simulink model "V2X_Core_SRI_coding_rate_symbol"  (R2023b)
settings: Solver=ode23tb  StartTime=0.0  StopTime=50  MaxStep=1e-2  RelTol=1e-3  AbsTol=1e-3
StopFcn:
  | run('saving.m')
values from neighbouring files (symbols this model uses):
  b = 1.6    [a2024_v2x_matlab_6veh.m]
  m = 2000    [a2024_v2x_matlab_6veh.m]
  mEgo = 1500    [a2024_v2x_matlab_6veh.m]
  Mode = 1    [a2024_v2x_matlab_6veh.m]    (also in v2x_matlab.m; v2x_matlabV2.m; v2x_matlab_6veh.m; v2x_matlab_R.m)
  RefSpeed = 90/3.6    (= 25)    [v2x_matlabV2.m]    (also in v2x_matlab_R.m)
  RelDistThreshold = 300    [v2x_matlabV2.m]    (also in v2x_matlab_R.m)
  s = RandStream("dsfmt19937","Seed",15)    [v2x_matlab.m]
  sampleTime = 0.1    [a2024_v2x_matlab_6veh.m]    (also in v2x_matlab.m; v2x_matlabV2.m; v2x_matlab_6veh.m; v2x_matlab_R.m)
  waypoints = [egoWP(:,2) egoWP(:,1), zeroforwp]    [a2024_v2x_matlab_6veh.m]    (also in misc.m = data.data.ActorSpecifications(1,1).Waypoints(:,[1,2]); v2x_matlab.m = data.data.ActorSpecifications(1,1).Waypoints(:,[1,2]); v2x_matlabV2.m = [5 -1.6 0; v2x_matlab_R.m = [5 -1.6 0)
  ZeroActors = struct(     'ActorID',0,     'Position', [1000 1000 1000],      'Velocity', [0 0 0],      'Roll', 0,      'Pitch', 0,      'Yaw', 0,      'AngularVelocity', [0 0 0])    [v2x_matlabV2.m]    (also in v2x_matlab_R.m)
undefined symbols (not defined in the file or in its folder): Battery, Brakes, Control, DiscIntNeverNeededParam, doppler, Drivetrain, ElectricMotor, Env, FB_flag, Init, SNR_value_list, Vehicle, Wheels
libraries: simulink x45, commofdm x29, commdigbbndam3 x15, commchan3 x14, simulink_extras x13, commcnvcod2 x12, commdigbbndpm3 x11, commblkintrlv2 x10, dspmathops x6, sharedtransform x6, autolibutils x6, autolibsharedcoupling x4
(part 7 of 8)

== matlab function V2X_Core_SRI_coding_rate_symbol/Subsystem2/MATLAB Function1 ==
  data: busActors3Test1 input; Actor output int16 size=15; VehicleID input; VehicleData output Bus: Actors; EgoData input Bus: Actors; counter output
  events: trigger input RISING_EDGE_EVENT
function [Actor, VehicleData, counter]  = convBus2IntVector(busActors3Test1, VehicleID, EgoData)

% Data extracted from actorss bus

%ActorId = BusActors1Actors.Actors(ActorID).ActorID(1:1);
numActors = busActors3Test1.NumActors;
%time = busActors3Test1.Time;
time = busActors3Test1.Time;

ActorID = VehicleID;

posX = busActors3Test1.Actors(ActorID).Position(1:1);
posY = busActors3Test1.Actors(ActorID).Position(2:2);
posZ = busActors3Test1.Actors(ActorID).Position(3:3);
vPos = [posX posY posZ];

vX = busActors3Test1.Actors(ActorID).Velocity(1:1);
vY = busActors3Test1.Actors(ActorID).Velocity(2:2);
vZ = busActors3Test1.Actors(ActorID).Velocity(3:3);

roll = busActors3Test1.Actors(ActorID).Roll(1:1);
pitch = busActors3Test1.Actors(ActorID).Pitch(1:1);
yaw = busActors3Test1.Actors(ActorID).Yaw(1:1);


angularVelocityX = busActors3Test1.Actors(ActorID).AngularVelocity(1:1);
angularVelocityY = busActors3Test1.Actors(ActorID).AngularVelocity(2:2);
angularVelocityZ = busActors3Test1.Actors(ActorID).AngularVelocity(3:3);

VehicleData = busActors3Test1.Actors(ActorID);


%% Converting the data

ActorID = int16(ActorID);

posMultip = 10;
posX = int16(round(posMultip*posX));
posY = int16(round(posMultip*posY));
posZ = int16(round(posMultip*posZ));

velMultip = 50;
vX = int16(round(velMultip * vX));
vY = int16(round(velMultip * vY));
vZ = int16(round(velMultip * vZ));

rpyMultip = 50;
roll = int16(round(rpyMultip * roll));
pitch = int16(round(rpyMultip * pitch));
yaw = int16(round(rpyMultip * yaw));

angvelMultip = 50;
angularVelocityX = int16(round(angvelMultip * angularVelocityX));
angularVelocityY = int16(round(angvelMultip * angularVelocityY));
angularVelocityZ = int16(round(angvelMultip * angularVelocityZ));


% Output vector
%zerosVector = zeros(9,1);

intVector = [numActors; time; ActorID; posX; posY; posZ; vX; vY; vZ; roll; pitch; yaw; angularVelocityX; angularVelocityY; angularVelocityZ];



%% Pathloss (freespace)

EgoPos = EgoData.Position;
dist = norm(vPos - EgoPos);

fc = 5.9*10^9;  % Carrier frequency
lambda = physconst('LightSpeed')/fc;

PL = fspl(dist, lambda);

Pt_dBm = 33;    % [dBm] Transmission power; maximum permissible transmit power level
sigma = rand(1) + 3.2;  % [3.7 +- 0.5] Variance of the shadowing effect in the wireless communication channel
                        % shadowing follows a log-normal random distribution
X = randn(1);       % random variable following a normal distribution with mean 0 and standard deviation 1
SH = sigma * X;

Pr = Pt_dBm - PL - SH;

P_SEN = -40;

ZeroActors = int16(zeros(15,1));

persistent prev_value;
if isempty(prev_value)
    prev_value = ZeroActors; % Initialize to a default value
end

if Pr > P_SEN
    Actor = intVector;
    prev_value = intVector;
else
    Actor = prev_value;
end


%% Packet counter
counter = 0;

if (Pr > P_SEN)
    counter = counter + 1;
end


end

== matlab function V2X_Core_SRI_coding_rate_symbol/VehicleDynamic/MATLAB Function1 ==
  data: RefSpeed input; RefSpeedMax output size=1; v_HV input; v_RV input; pdr input; lat input; sri_target input; sri_val output; RelDist input; Headway output
function [RefSpeedMax, sri_val, Headway] = calculate_SRI_max_speed(RefSpeed, v_HV, v_RV, pdr, lat, sri_target, RelDist)

    %V_HV_UPPER_LIMIT = 1.0
    %V_HV_LOWER_LIMIT = 0.0
    % SRI_TARGET = 0.1;
    DEFAULT_HV_SPEED = 190 / 3.6; % in m/s
    DEFAULT_RV_SPEED =  190 / 3.6; % in m/s


    pdr_normalized = pdr / 100;
    lat_normalized = lat / 1000;
    v_HV_normalized = v_HV / DEFAULT_HV_SPEED;
    v_RV_normalized = v_RV / DEFAULT_RV_SPEED;
    
    if abs(v_HV) < 0.001
        Speed_reciproc = 0;
    else
        Speed_reciproc = 1/v_HV;
    end

    Headway = RelDist*Speed_reciproc;
    if Headway > 50
        Headway = 50;
    end



    if v_RV-1 > v_HV || pdr < 0.1
        RefSpeedMax = RefSpeed;
        sri_val = -1;
    else
        sri_val = SRI_value(v_HV_normalized,v_RV_normalized, pdr_normalized, lat_normalized);
        if sri_val <= sri_target
            RefSpeedMax = RefSpeed;
        else
            lb0 = 0.0;
            ub0 = v_HV_normalized;
            x0 = 1.0;
            %value_bounds = Bounds([V_HV_LOWER_LIMIT],[v_HV_normalized])
            opts = optimoptions('fmincon','Algorithm','sqp');
            sri_err_fun = @(v_HV_norm) abs(SRI_value(v_HV_norm, v_RV_normalized, pdr_normalized, lat_normalized) - sri_target); 
            v_HV_max_normalized = fmincon(sri_err_fun, x0,[], [],[],[], lb0, ub0, [], opts);
            %res = minimize(fun=SRI_target_function, x0=[1.0], bounds=value_bounds, args=(v_RV_normalized, pdr_normalized, lat_normalized, sri_target))
            %v_HV_max_normalized = res.x[0];
            if Headway < 1.3
                RefSpeedMax = v_RV;
            else
                RefSpeedMax = v_HV_max_normalized*DEFAULT_HV_SPEED; % in m/s
            end
        end
    end

end
function sri_value = SRI_value(v_HV_norm, v_RV_norm, pdr_norm, lat_norm)

    OLSparams = [0.1283, -0.0089, -0.2621, -0.0181, 0.6640, -0.0156, -0.2030, -1.1130, 0.3615, 0.1294, 0.5597, 0.1044, 0.0613, -0.5524, 0.0934];
    sri_value =   OLSparams(1) ...
                + OLSparams(2)  * v_HV_norm ...
                + OLSparams(3)  * v_RV_norm ...
                + OLSparams(4)  * pdr_norm ...
                + OLSparams(5)  * v_HV_norm^2 ...
                + OLSparams(6)  * v_RV_norm^2 ...
                + OLSparams(7)  * v_RV_norm * pdr_norm ...
                + OLSparams(8)  * pdr_norm * (v_HV_norm^2) ...
                + OLSparams(9)  * pdr_norm * (v_RV_norm^2) ...
                + OLSparams(10) * lat_norm * (v_HV_norm^2) ...
                + OLSparams(11) * (v_HV_norm^2) * (pdr_norm^2) ...
                + OLSparams(12) * v_HV_norm * v_RV_norm * lat_norm ...
                + OLSparams(13) * v_RV_norm * pdr_norm * lat_norm ...
                + OLSparams(14) * v_RV_norm * lat_norm * (v_HV_norm^2)...
                + OLSparams(15) * lat_norm * (v_HV_norm^2) * (v_RV_norm^2);
end


% % 
% % v_HV_0 = 0.0;
% % SRI_target = 0.5;
% % v_RV = v_RV_original / (50.0/3.6);
% % 
% % OLSparams = [0.1283, -0.0089, -0.2621, -0.0181, 0.6640, -0.0156, -0.2030, -1.1130, 0.3615, 0.1294, 0.5597, 0.1044, 0.0613, -0.5524, 0.0934];
% % 
% % 
% % SRI = @(v_HV) abs(OLSparams(1) ...
% %                 + OLSparams(2) * PDR ...
% %                 + OLSparams(3) * LAT ...
% %                 + OLSparams(4) * v_HV ...
% %                 + OLSparams(5) * v_HV^2 ...
% %                 + OLSparams(6) * PDR * v_HV ...
% %                 + OLSparams(7) * PDR * v_RV ...
% %                 + OLSparams(8) * v_HV * v_RV^2 ...
% %                 + OLSparams(9) * v_RV * v_HV^2 ...
% %                 + OLSparams(10) * PDR * v_RV * v_HV^2 ...
% %                 + OLSparams(11) * PDR^2 * v_HV * v_RV^2 ...
% %                 + OLSparams(12) * PDR^2 * v_HV^2 * v_RV ...
% %                 + OLSparams(13) * PDR^2 * v_HV^2*v_RV^2 ...
% %                 - SRI_target);
% %  v_HV = fminsearch(SRI, v_HV_0) * 130.0/3.6;
% % end

== matlab function V2X_Core_SRI_coding_rate_symbol/DSRC/Subsystem3/3//4 64 QAM/MATLAB Function3 ==
  settings: updateMethod=DISCRETE
  data: input input; output output
function output = removeZeros(input)

output = input(1:40,:,:);

end

== matlab function V2X_Core_SRI_coding_rate_symbol/DSRC/Subsystem4/MATLAB Function1 ==
  settings: sampleTime=inherited
  data: busActors3Test1 input; Actor output int16 size=15; VehicleID input; VehicleData output Bus: Actors; EgoData input Bus: Actors; counter_out output; SNR output; Pr output
  events: trigger input RISING_EDGE_EVENT
function [Actor, VehicleData, counter_out, SNR, Pr]  = convBus2IntVector(busActors3Test1, VehicleID, EgoData)

% Data extracted from actorss bus

%ActorId = BusActors1Actors.Actors(ActorID).ActorID(1:1);
numActors = busActors3Test1.NumActors;
%time = busActors3Test1.Time;
time = busActors3Test1.Time;

ActorID = VehicleID;

posX = busActors3Test1.Actors(ActorID).Position(1:1);
posY = busActors3Test1.Actors(ActorID).Position(2:2);
posZ = busActors3Test1.Actors(ActorID).Position(3:3);
vPos = [posX posY posZ];

vX = busActors3Test1.Actors(ActorID).Velocity(1:1);
vY = busActors3Test1.Actors(ActorID).Velocity(2:2);
vZ = busActors3Test1.Actors(ActorID).Velocity(3:3);

roll = busActors3Test1.Actors(ActorID).Roll(1:1);
pitch = busActors3Test1.Actors(ActorID).Pitch(1:1);
yaw = busActors3Test1.Actors(ActorID).Yaw(1:1);


angularVelocityX = busActors3Test1.Actors(ActorID).AngularVelocity(1:1);
angularVelocityY = busActors3Test1.Actors(ActorID).AngularVelocity(2:2);
angularVelocityZ = busActors3Test1.Actors(ActorID).AngularVelocity(3:3);

VehicleData = busActors3Test1.Actors(VehicleID);


%% Converting the data

ActorID = int16(ActorID);

posMultip = 10;
posX = int16(round(posMultip*posX));
posY = int16(round(posMultip*posY));
posZ = int16(round(posMultip*posZ));

velMultip = 50;
vX = int16(round(velMultip * vX));
vY = int16(round(velMultip * vY));
vZ = int16(round(velMultip * vZ));

rpyMultip = 50;
roll = int16(round(rpyMultip * roll));
pitch = int16(round(rpyMultip * pitch));
yaw = int16(round(rpyMultip * yaw));

angvelMultip = 50;
angularVelocityX = int16(round(angvelMultip * angularVelocityX));
angularVelocityY = int16(round(angvelMultip * angularVelocityY));
angularVelocityZ = int16(round(angvelMultip * angularVelocityZ));


% Output vector
%zerosVector = zeros(9,1);

intVector = [numActors; time; ActorID; posX; posY; posZ; vX; vY; vZ; roll; pitch; yaw; angularVelocityX; angularVelocityY; angularVelocityZ];


%% Pathloss (freespace)

EgoPos = EgoData.Position;
dist = norm(vPos - EgoPos);

fc = 5.9e9;  % Carrier frequency
lambda = (physconst('LightSpeed'))/fc;

PL = fspl(dist, lambda);

Pt_dBm = 33;    % [dBm] Transmission power; maximum permissible transmit power level
Pt_dbW = Pt_dBm - 30;
sigma = rand(1) + 3.2;  % [3.7 +- 0.5] Variance of the shadowing effect in the wireless communication channel
                        % shadowing follows a log-normal random distribution
X = 2*rand(1)-1;      % random variable following a normal distribution with mean 0 and standard deviation 1
SH = sigma * X;

% h_T = 1;
% h_R = 1;
% dF =  (4*h_T*h_R)/lambda
% lambda1 = 1.61; % Pathloss exponent LOS
% lambda2 = 1.85; % Pathloss exponent NLOS

Pr = Pt_dBm - PL - SH; 

% l1 = 10*lambda1*log(dF)
% l2 = 10*lambda2*log(dist/dF)
% Pr = Prt - l1 - l2 + SH;

P_SEN = -60;

%ZeroActors = int16(zeros(15,1));
% 
% counter = 0;
% storedPacket = int16(nan(15,1));
% 
% if Pr > P_SEN
%     Actor = intVector;
%     storedPacket = intVector;
%     counter = 0;
% elseif counter < 10
%     Actor = storedPacket;
%     counter = counter + 1;
% end


%disp(storedPacket)


% persistent prev_value;
% if isempty(prev_value)
%     prev_value = int16(nan(15,1)); % Initialize to a default value
% end
% 
% if Pr > P_SEN
%     Actor = intVector;
%     prev_value = intVector;
%     counter = 0;
% elseif counter < 1
%     Actor = prev_value;
%     counter = counter + 1;
% end

Actor = intVector;
%% SNR
bandwidth = 10e6;
F = 6; % [dB] Noise figure
k = physconst('Boltzmann'); % Boltzmann állandó
T = 300; % [K] Abszolút hőmérséklet

N0 = bandwidth *k*T;
N0dbm = 10 * log10(1000*N0);
N0dbW = N0dbm - 30; 
%N0 = -99;
SNR = Pr - N0dbm;
%signalpower = Pr;s


%% Packet counter
persistent counter
if isempty(counter)
    counter = 0;
end

if (Pr > P_SEN)
    counter = counter + 1;
end

counter_out = counter;
end

== matlab function V2X_Core_SRI_coding_rate_symbol/DSRC/Subsystem4/MATLAB Function2 ==
  settings: updateMethod=DISCRETE  sampleTime=sampleTime
  data: modulated input; signal output; SNR input
function signal = PRO_error(modulated, SNR)

signal = awgn(modulated,SNR);

== matlab function V2X_Core_SRI_coding_rate_symbol/Channel/MATLAB Function1 ==
  data: Actors output Bus: Actors; ActorsIn input; Positions output; Distances output; Ego input
function [Actors, Positions, Distances] = SelectActor(ActorsIn, Ego)

EgoActor = Ego;
Actors = ActorsIn.Actors;


% Separating
Lead = ActorsIn.Actors(1);
Interfering = ActorsIn.Actors(3);
Threshold = ActorsIn.Actors(2);

% Distances
EgoPos = Ego.Position';
LeadPos = Lead.Position';
InterferingPos = Interfering.Position';
ThresholdPos = Threshold.Position';

Positions = [EgoPos LeadPos InterferingPos ThresholdPos];

%EgoDists
EgoDist = [norm(EgoPos-EgoPos);
            norm(EgoPos-LeadPos);
            norm(EgoPos-InterferingPos);
            norm(EgoPos-ThresholdPos)];

%LeadDists
LeadDist = [norm(LeadPos-EgoPos);
            norm(LeadPos-LeadPos);
            norm(LeadPos-InterferingPos);
            norm(LeadPos-ThresholdPos)];

%InterferringDists
InterferringDist = [norm(InterferingPos-EgoPos);
                    norm(InterferingPos-LeadPos);
                    norm(InterferingPos-InterferingPos);
                    norm(InterferingPos-ThresholdPos)];

% ThresholdDists
ThresholdDist = [norm(ThresholdPos-EgoPos);
                norm(ThresholdPos-LeadPos);
                norm(ThresholdPos-InterferingPos);
                norm(ThresholdPos-ThresholdPos)];


Distances = [EgoDist, LeadDist, InterferringDist, ThresholdDist] ;

end

== matlab function V2X_Core_SRI_coding_rate_symbol/DSRC/Subsystem5/MATLAB Function1 ==
  settings: sampleTime=inherited
  data: busActors3Test1 input; Actor output int16 size=15; VehicleID input; VehicleData output Bus: Actors; EgoData input Bus: Actors; counter_out output; SNR output; Pr output
  events: trigger input RISING_EDGE_EVENT
function [Actor, VehicleData, counter_out, SNR, Pr]  = convBus2IntVector(busActors3Test1, VehicleID, EgoData)

% Data extracted from actorss bus

%ActorId = BusActors1Actors.Actors(ActorID).ActorID(1:1);
numActors = busActors3Test1.NumActors;
%time = busActors3Test1.Time;
time = busActors3Test1.Time;

ActorID = VehicleID;

posX = busActors3Test1.Actors(ActorID).Position(1:1);
posY = busActors3Test1.Actors(ActorID).Position(2:2);
posZ = busActors3Test1.Actors(ActorID).Position(3:3);
vPos = [posX posY posZ];

vX = busActors3Test1.Actors(ActorID).Velocity(1:1);
vY = busActors3Test1.Actors(ActorID).Velocity(2:2);
vZ = busActors3Test1.Actors(ActorID).Velocity(3:3);

roll = busActors3Test1.Actors(ActorID).Roll(1:1);
pitch = busActors3Test1.Actors(ActorID).Pitch(1:1);
yaw = busActors3Test1.Actors(ActorID).Yaw(1:1);


angularVelocityX = busActors3Test1.Actors(ActorID).AngularVelocity(1:1);
angularVelocityY = busActors3Test1.Actors(ActorID).AngularVelocity(2:2);
angularVelocityZ = busActors3Test1.Actors(ActorID).AngularVelocity(3:3);

VehicleData = busActors3Test1.Actors(VehicleID);


%% Converting the data

ActorID = int16(ActorID);

posMultip = 10;
posX = int16(round(posMultip*posX));
posY = int16(round(posMultip*posY));
posZ = int16(round(posMultip*posZ));

velMultip = 50;
vX = int16(round(velMultip * vX));
vY = int16(round(velMultip * vY));
vZ = int16(round(velMultip * vZ));

rpyMultip = 50;
roll = int16(round(rpyMultip * roll));
pitch = int16(round(rpyMultip * pitch));
yaw = int16(round(rpyMultip * yaw));

angvelMultip = 50;
angularVelocityX = int16(round(angvelMultip * angularVelocityX));
angularVelocityY = int16(round(angvelMultip * angularVelocityY));
angularVelocityZ = int16(round(angvelMultip * angularVelocityZ));


% Output vector
%zerosVector = zeros(9,1);

intVector = [numActors; time; ActorID; posX; posY; posZ; vX; vY; vZ; roll; pitch; yaw; angularVelocityX; angularVelocityY; angularVelocityZ];


%% Pathloss (freespace)

EgoPos = EgoData.Position;
dist = norm(vPos - EgoPos);

fc = 5.9e9;  % Carrier frequency
lambda = (physconst('LightSpeed'))/fc;

PL = fspl(dist, lambda);

Pt_dBm = 33;    % [dBm] Transmission power; maximum permissible transmit power level
Pt_dbW = Pt_dBm - 30;
sigma = rand(1) + 3.2;  % [3.7 +- 0.5] Variance of the shadowing effect in the wireless communication channel
                        % shadowing follows a log-normal random distribution
X = 2*rand(1)-1;      % random variable following a normal distribution with mean 0 and standard deviation 1
SH = sigma * X;

% h_T = 1;
% h_R = 1;
% dF =  (4*h_T*h_R)/lambda
% lambda1 = 1.61; % Pathloss exponent LOS
% lambda2 = 1.85; % Pathloss exponent NLOS

Pr = Pt_dBm - PL - SH; 

% l1 = 10*lambda1*log(dF)
% l2 = 10*lambda2*log(dist/dF)
% Pr = Prt - l1 - l2 + SH;

P_SEN = -60;

%ZeroActors = int16(zeros(15,1));
% 
% counter = 0;
% storedPacket = int16(nan(15,1));
% 
% if Pr > P_SEN
%     Actor = intVector;
%     storedPacket = intVector;
%     counter = 0;
% elseif counter < 10
%     Actor = storedPacket;
%     counter = counter + 1;
% end


%disp(storedPacket)


% persistent prev_value;
% if isempty(prev_value)
%     prev_value = int16(nan(15,1)); % Initialize to a default value
% end
% 
% if Pr > P_SEN
%     Actor = intVector;
%     prev_value = intVector;
%     counter = 0;
% elseif counter < 1
%     Actor = prev_value;
%     counter = counter + 1;
% end

Actor = intVector;
%% SNR
bandwidth = 10e6;
F = 6; % [dB] Noise figure
k = physconst('Boltzmann'); % Boltzmann állandó
T = 300; % [K] Abszolút hőmérséklet

N0 = bandwidth *k*T;
N0dbm = 10 * log10(1000*N0);
N0dbW = N0dbm - 30; 
%N0 = -99;
SNR = Pr - N0dbm;
%signalpower = Pr;s


%% Packet counter
persistent counter
if isempty(counter)
    counter = 0;
end

if (Pr > P_SEN)
    counter = counter + 1;
end

counter_out = counter;
end

== matlab function V2X_Core_SRI_coding_rate_symbol/DSRC/Subsystem5/MATLAB Function2 ==
  settings: updateMethod=DISCRETE  sampleTime=sampleTime
  data: modulated input; signal output; SNR input
function signal = PRO_error(modulated, SNR)

signal = awgn(modulated,SNR);

== matlab function V2X_Core_SRI_coding_rate_symbol/Channel/MATLAB Function9 ==
  data: Ego input; Actors input Bus: Actors; LeadActor output Bus: Actors size=1; InterferingActor output Bus: Actors size=1; ThresholdActor output Bus: Actors size=1; PSR output; Positions input; ZeroActors input
function [LeadActor,InterferingActor,ThresholdActor,PSR] = SEN_PSR(Ego, Actors, Positions, ZeroActors)
coder.extrinsic('Simulink.Bus')

%% Extract data
Lead = Actors(1);
Interfering = Actors(2);
Threshold = Actors(3);

EgoPos = Positions(:,1);
LeadPos = Positions(:,2);
InterferingPos = Positions(:,3);
ThresholdPos = Positions(:,4);

%% Calculating distances
de_lead = norm(LeadPos - EgoPos);                % Ego-Lead Distance
de_interfering = norm(InterferingPos - EgoPos);  % Ego-Interferring Distance
de_threshold = norm(ThresholdPos  - EgoPos);     % Ego-Threshold distance

dl_interfering = norm(InterferingPos - LeadPos);
dl_threshold = norm(ThresholdPos - LeadPos);

di_threshold = norm(ThresholdPos - InterferingPos);

%% Pathloss (freespace)
fc = 5.9*10^9;  % Carrier frequency
lambda = physconst('LightSpeed')/fc;

PL_EL = fspl(de_lead, lambda);
PL_EI = fspl(de_interfering, lambda);
PL_ET = fspl(de_threshold, lambda);

PL_LI = fspl(dl_interfering, lambda);
PL_LT = fspl(dl_threshold, lambda);

PL_IT = fspl(di_threshold, lambda);


% Transmission Power (Pt)
Pt_dBm = 33;    % [dBm] Transmission power; maximum permissible transmit power level
%Pt_dBw = Pt_dBm - 30; % [dBw]
%Pt_watts = (10 .^ (dBm / 10))/1000;  % Transmission power in W

sigma = rand(1) + 3.2;  % [3.7 +- 0.5] Variance of the shadowing effect in the wireless communication channel
                        % shadowing follows a log-normal random distribution
X = randn(1);       % random variable following a normal distribution with mean 0 and standard deviation 1
SH = sigma * X;
Pr_EL = Pt_dBm - PL_EL - SH; 
Pr_EI = Pt_dBm - PL_EI - SH;
Pr_ET = Pt_dBm - PL_ET - SH;

Pr_LI = Pt_dBm - PL_LI  - SH;
Pr_LT = Pt_dBm - PL_LT  - SH;

Pr_IT = Pt_dBm - PL_IT  - SH;


P_SEN = -60;  % [dBm] Sensing threshold
% P_SEN_dBW = P_SEN + 30;

% Lead
persistent prev_value_lead;
if isempty(prev_value_lead)
    prev_value_lead = ZeroActors; % Initialize to a default value
end

if Pr_EL > P_SEN
    LeadActor = Lead;
    prev_value_lead = Lead;
else
    LeadActor = prev_value_lead;
end

% Interfering
%InterferingActorOut = struct;

persistent prev_value_int;
if isempty(prev_value_int)
    prev_value_int = ZeroActors; % Initialize to a default value
end

if Pr_EI > P_SEN
    InterferingActor = Interfering;
    prev_value_int = Interfering;
else
    InterferingActor = prev_value_int;
end

% Threshold
persistent prev_value_thr;


if isempty(prev_value_thr)
    prev_value_thr = ZeroActors; % Initialize to a default value
end

if Pr_ET > P_SEN
    ThresholdActor = Threshold;
    prev_value_thr = Threshold;
else
    ThresholdActor = prev_value_thr;
end


%% PSR 
sigmasqrt2 = sigma * sqrt(2);

% Ego - Lead
deltaPtSEN_EL = Pt_dBm - PL_EL - P_SEN;
delta_SEN_EL = 0.5*(1-erf(deltaPtSEN_EL/sigmasqrt2));
PSR_EL = 1-delta_SEN_EL;

% Ego - Interfering
deltaPtSEN_EI = Pt_dBm - PL_EI - P_SEN;
delta_SEN_EI = 0.5*(1-erf(deltaPtSEN_EI/sigmasqrt2));
PSR_EI = 1-delta_SEN_EI;

% Ego - Threshold
deltaPtSEN_ET = Pt_dBm - PL_ET - P_SEN;
delta_SEN_ET = 0.5*(1-erf(deltaPtSEN_ET/sigmasqrt2));
PSR_ET = 1-delta_SEN_ET;

% Lead - Interfering
deltaPtSEN_LI = Pt_dBm - PL_LI - P_SEN;
delta_SEN_LI = 0.5*(1-erf(deltaPtSEN_LI/sigmasqrt2));
PSR_LI = 1-delta_SEN_LI;

% Lead - Threshold
deltaPtSEN_LT = Pt_dBm - PL_LT - P_SEN;
delta_SEN_LT = 0.5*(1-erf(deltaPtSEN_LT/sigmasqrt2));
PSR_LT = 1-delta_SEN_LT;

% Interfering - Threshold;
deltaPtSEN_IT = Pt_dBm - PL_IT - P_SEN;
delta_SEN_IT = 0.5*(1-erf(deltaPtSEN_IT/sigmasqrt2));
PSR_IT = 1-delta_SEN_IT;


PSR = [PSR_EL PSR_EI PSR_ET PSR_LI PSR_LT PSR_IT];

end

== matlab function V2X_Core_SRI_coding_rate_symbol/Channel/MATLAB Function4 ==
  data: PSR input; CBR output
function CBR = CBR(PSR)

lambda = (1/0.01)*3;            % Packets/second
T = 0.008;                      % Packet duration


beta = 4*4.7/400;   % Traffic density (vehicle/meter)

load_ir = lambda * T * PSR;

% CBR upper bound:
CBR_u = beta * sum(load_ir);    % distance between vehicle vi and the ego vehicle
                                % upper bound, because it does not take into account packet collisions
p1 = -0.2481;
p2 = 0.913;
p3 = 0.003844;

CBR = p1*CBR_u^2 + p2*CBR_u + p3

end

== matlab function V2X_Core_SRI_coding_rate_symbol/Ego trajectory ==
  settings: updateMethod=DISCRETE  sampleTime=sampleTime
  data: EgoFdbX input; EgoFdbY input; LongRef output; LatRef output; YawRef output; waypoints input
function [LongRef, LatRef, YawRef] = generateTrajectory(EgoFdbX, EgoFdbY, waypoints)

LongFdb = EgoFdbX;
LatFdb = EgoFdbY;
EgoFdb= [LongFdb, LatFdb]; % Ego feedback positions norm

% waypoints = [-104.6000, 6.6000, deg2rad(2.9993);
%             54.7000, -14.8000, deg2rad(-29.0375);
%             91.4000, -42.6000, deg2rad(-44.2776);
%             163.6000, -148.6000, deg2rad(-61.4646)];





count = 1;

min_distance = inf;

for i = 1:size(waypoints, 1)
    RefPose = waypoints(i,1:2);
    distance = norm(RefPose - EgoFdb);

    if abs(distance) < min_distance
        min_distance = abs(distance);
        count = i;
    end
end


if count > size(waypoints, 1)
    count = size(waypoints, 1);  % Ensure count doesn't exceed the number of rows in waypoints
end


LongRef = waypoints(count,1);
LatRef = waypoints(count,2);
YawRef = waypoints(count,3);
Output = [LongRef, LatRef, YawRef];
end


% while count <= size(waypoints, 1)
%     RefPosenorm = norm(waypoints(count,1:2));
%     if EgoFdbnorm < RefPosenorm
%         break;
%     else
%         count = count + 1;
%     end
% end
% 
% if count > size(waypoints, 1)
%     count = size(waypoints, 1);  
% end
% 
% RefPose = waypoints(count,:);
% end

% if 0 <= timevector < 1
%     RefPose = waypoints(1,:);
% elseif 1 <= timevector < 2
%     RefPose = waypoints(2,:);
% elseif 2 <= timevector < 3
%     RefPose = waypoints(3,:);
% elseif 3 <= timevector < 4
%     RefPose = waypoints(4,:);
% elseif 4 <= timevector < 5
%     RefPose = waypoints(5,:);
% elseif 5 <= timevector < 6
%     RefPose = waypoints(6,:);
% elseif 6 <= timevector < 7
%     RefPose = waypoints(7,:);
% elseif 7 <= timevector < 8
%     RefPose = waypoints(8,:);
% elseif 8 <= timevector < 9
%     RefPose = waypoints(9,:);
% elseif 9 <= timevector < 10
%     RefPose = waypoints(10,:);
% elseif 10 <= timevector < 11
%     RefPose = waypoints(11,:);
% end
% 
% end

== stateflow chart V2X_Core_SRI_coding_rate_symbol/VehicleDynamic/FiveSteteABS-TCS/ABSCtrlForEach/For Each Subsystem/ABSForEachWheel ==
  state ABSOff
    entry:
    PbOutput = Pref;
    Flag = 0;
    during:
    PbOutput = Pref;
  state Normal
    entry:
    PbOutput = Pref;
    Flag = 0;
    during:
    PbOutput = Pref;
  state ABSOn
    state Phase1
      entry:
      PbOutput = v1;
      Flag = 1;
    state Phase5
      entry:
      PbOutput = v5;
      Flag = 5;
    state Phase2
      entry:
      PbOutput = 0;
      Flag = 2;
    state Phase4
      entry:
      PbOutput = 0;
      Flag = 4;
    state Phase3
      entry:
      PbOutput = v4;
      Flag = 3;
    (default) -> Phase1
    Phase5 -> Phase1 : [e2 < a2]
    Phase1 -> Phase2 : [e2 >= b]
    Phase4 -> Phase5 : [e2 <= a1]
    Phase2 -> Phase3 : [e2 >= A]
    Phase3 -> Phase4 : [e2 < A]
  (default) -> ABSOff
  ABSOn -> ABSOff : [abs(VehSpd) < 0.1 || Pref <= 0]
  Normal -> ABSOff [order 2] : [Pref <= 0]
  ABSOff -> Normal : [Pref > 0 && e2 < a2]
  Normal -> ABSOn [order 1] : [e1 < 0]
  data: e1 input; e2 input; PbOutput output; Flag output; b parameter; v1 parameter; v4 parameter; v5 parameter; A parameter; a2 parameter; a1 parameter; Pref input; VehSpd input

== stateflow chart V2X_Core_SRI_coding_rate_symbol/VehicleDynamic/FiveSteteABS-TCS/TCSCtrlForEach/For Each Subsystem/ABSForEachWheel ==
  state TCSOff
    entry:
    PbOutput = 0;
    Flag = 0;
    during:
    PbOutput = 0;
  state Normal
    entry:
    PbOutput = 0;
    Flag = 0;
    during:
    PbOutput = 0;
  state TCSOn
    state Phase1
      entry:
      PbOutput = v1;
      Flag = 1;
    state Phase5
      entry:
      PbOutput = v5;
      Flag = 5;
    state Phase2
      entry:
      PbOutput = 0;
      Flag = 2;
    state Phase4
      entry:
      PbOutput = 0;
      Flag = 4;
    state Phase3
      entry:
      PbOutput = v4;
      Flag = 3;
    (default) -> Phase1
    Phase5 -> Phase1 : [e2 > a2]
    Phase1 -> Phase2 : [e2 <= b]
    Phase4 -> Phase5 : [e2 >= a1]
    Phase2 -> Phase3 : [e2 <= A]
    Phase3 -> Phase4 : [e2 > A]
  (default) -> TCSOff
  TCSOn -> TCSOff : [Pb <= 0 || AccelFdbk <= 0.2|| e1<0.1]
  Normal -> TCSOff [order 2] : [AccelFdbk <= 0]
  TCSOff -> Normal : [AccelFdbk > 0 && e2 > a2 && Enb > 0.3]
  Normal -> TCSOn [order 1] : [e1 > 0]
  data: e1 input; e2 input; PbOutput output; Flag output; b parameter; v1 parameter; v4 parameter; v5 parameter; A parameter; a2 parameter; a1 parameter; AccelFdbk input; Enb input; Pb input

== matlab function V2X_Core_SRI_coding_rate_symbol/MATLAB Function6 ==
  settings: updateMethod=DISCRETE  sampleTime=sampleTime
  data: xdotin input; y output
function y = initialVelocity(xdotin)

if isempty(xdotin) == true
    y = 16;
elseif xdotin == 0
    y = 16;
else
    y = abs(xdotin);
end

end

== matlab function V2X_Core_SRI_coding_rate_symbol/MATLAB Function3 ==
  settings: updateMethod=DISCRETE  sampleTime=sampleTime
  data: EgoActor input; busActors3Test1 input; Dist output
function Dist = fcn(EgoActor, busActors3Test1)

EgoPos = EgoActor.Position;

Position1  = double(busActors3Test1.Actors(1).Position);
Position2  = double(busActors3Test1.Actors(2).Position);
Position3  = double(busActors3Test1.Actors(3).Position);
Position4  = double(busActors3Test1.Actors(4).Position);
Position5  = double(busActors3Test1.Actors(5).Position);

Dist1 = norm(EgoPos-Position1);
Dist2 = norm(EgoPos-Position2);
Dist3 = norm(EgoPos-Position3);
Dist4 = norm(EgoPos-Position4);
Dist5 = norm(EgoPos-Position5);

Dist = [Dist1; Dist2; Dist3; Dist4; Dist5]

end

== matlab function V2X_Core_SRI_coding_rate_symbol/Perception/MATLAB Function7 ==
  settings: updateMethod=DISCRETE  sampleTime=sampleTime
  data: u input; RelVel output
function RelVel = fcn(u)

for i = 1:5
    RelVel = 0;
end

RelVel = u;

== matlab function V2X_Core_SRI_coding_rate_symbol/Perception/MATLAB Function8 ==
  settings: updateMethod=DISCRETE  sampleTime=sampleTime
  data: u input; RelDist output
function RelDist = fcn(u)

for i = 1:5
    RelDist = 9999;
end

RelDist = u;

== matlab function V2X_Core_SRI_coding_rate_symbol/VehicleDynamic/Suspension to Chasiss Transforms/Estimated Unsprung Mass Orientation ==
  data: angles output size=3; angleIn input size=3; GeomXYZ output size=3; GemoXYZIn input size=3; Ground input size=4; trackW parameter; wheelB parameter
function [angles,GeomXYZ]= three26(angleIn, GemoXYZIn, Ground,trackW, wheelB)%#codegen
coder.allowpcode('plain')
% Copyright 2018 The MathWorks, Inc.
[angles,GeomXYZ]= vdynthree2six(angleIn, GemoXYZIn, Ground,trackW, wheelB);

== matlab function V2X_Core_SRI_coding_rate_symbol/DSRC/Subsystem5/MATLAB Function3 ==
  settings: sampleTime=sampleTime
  data: input input; Actors output
function Actors = getRealValues(input) 

modulated = input;

NumActors = modulated(1,:);
Time = modulated(2,:);

ActorID = modulated(3,1);

posMultip = 10;  % 10
posX = (modulated(4,:)/posMultip);
posY = (modulated(5,:)/posMultip);
posZ = (modulated(6,:)/posMultip);

velMultip = 50;  % 50
vX = (modulated(7,:)/velMultip);
vY = (modulated(8,:)/velMultip);
vZ = (modulated(9,:)/velMultip);

rpyMultip = 50;  % 50
Roll = (modulated(10,:)/rpyMultip);
Pitch = (modulated(11,:)/rpyMultip);
Yaw = (modulated(12,:)/rpyMultip);

angvelMultip = 50;  % 50
angularVelocityX = (modulated(13,:)/angvelMultip);
angularVelocityY = (modulated(14,:)/angvelMultip);
angularVelocityZ = (modulated(15,:)/angvelMultip);

% Velocity = [vX vY vZ];
% Position = [posX posY posZ];
% AngularVelocity = [angularVelocityX; angularVelocityY; angularVelocityZ];


%Actors = [NumActors; Time; ActorID; Position; Velocity; Roll; Pitch; Yaw; AngularVelocity];
Actors = double([NumActors; Time; ActorID; posX; posY; posZ; vX; vY; vZ; Roll; Pitch; Yaw; angularVelocityX; angularVelocityY; angularVelocityZ]);


end

== matlab function V2X_Core_SRI_coding_rate_symbol/DSRC/Subsystem6/MATLAB Function1 ==
  settings: sampleTime=inherited
  data: busActors3Test1 input; Actor output int16 size=15; VehicleID input; VehicleData output Bus: Actors; EgoData input Bus: Actors; counter_out output; SNR output; Pr output
  events: trigger input RISING_EDGE_EVENT
function [Actor, VehicleData, counter_out, SNR, Pr]  = convBus2IntVector(busActors3Test1, VehicleID, EgoData)

% Data extracted from actorss bus

%ActorId = BusActors1Actors.Actors(ActorID).ActorID(1:1);
numActors = busActors3Test1.NumActors;
%time = busActors3Test1.Time;
time = busActors3Test1.Time;

ActorID = VehicleID;

posX = busActors3Test1.Actors(ActorID).Position(1:1);
posY = busActors3Test1.Actors(ActorID).Position(2:2);
posZ = busActors3Test1.Actors(ActorID).Position(3:3);
vPos = [posX posY posZ];

vX = busActors3Test1.Actors(ActorID).Velocity(1:1);
vY = busActors3Test1.Actors(ActorID).Velocity(2:2);
vZ = busActors3Test1.Actors(ActorID).Velocity(3:3);

roll = busActors3Test1.Actors(ActorID).Roll(1:1);
pitch = busActors3Test1.Actors(ActorID).Pitch(1:1);
yaw = busActors3Test1.Actors(ActorID).Yaw(1:1);


angularVelocityX = busActors3Test1.Actors(ActorID).AngularVelocity(1:1);
angularVelocityY = busActors3Test1.Actors(ActorID).AngularVelocity(2:2);
angularVelocityZ = busActors3Test1.Actors(ActorID).AngularVelocity(3:3);

VehicleData = busActors3Test1.Actors(VehicleID);


%% Converting the data

ActorID = int16(ActorID);

posMultip = 10;
posX = int16(round(posMultip*posX));
posY = int16(round(posMultip*posY));
posZ = int16(round(posMultip*posZ));

velMultip = 50;
vX = int16(round(velMultip * vX));
vY = int16(round(velMultip * vY));
vZ = int16(round(velMultip * vZ));

rpyMultip = 50;
roll = int16(round(rpyMultip * roll));
pitch = int16(round(rpyMultip * pitch));
yaw = int16(round(rpyMultip * yaw));

angvelMultip = 50;
angularVelocityX = int16(round(angvelMultip * angularVelocityX));
angularVelocityY = int16(round(angvelMultip * angularVelocityY));
angularVelocityZ = int16(round(angvelMultip * angularVelocityZ));


% Output vector
%zerosVector = zeros(9,1);

intVector = [numActors; time; ActorID; posX; posY; posZ; vX; vY; vZ; roll; pitch; yaw; angularVelocityX; angularVelocityY; angularVelocityZ];


%% Pathloss (freespace)

EgoPos = EgoData.Position;
dist = norm(vPos - EgoPos);

fc = 5.9e9;  % Carrier frequency
lambda = (physconst('LightSpeed'))/fc;

PL = fspl(dist, lambda);

Pt_dBm = 33;    % [dBm] Transmission power; maximum permissible transmit power level
Pt_dbW = Pt_dBm - 30;
sigma = rand(1) + 3.2;  % [3.7 +- 0.5] Variance of the shadowing effect in the wireless communication channel
                        % shadowing follows a log-normal random distribution
X = 2*rand(1)-1;      % random variable following a normal distribution with mean 0 and standard deviation 1
SH = sigma * X;

% h_T = 1;
% h_R = 1;
% dF =  (4*h_T*h_R)/lambda
% lambda1 = 1.61; % Pathloss exponent LOS
% lambda2 = 1.85; % Pathloss exponent NLOS

Pr = Pt_dBm - PL - SH; 

% l1 = 10*lambda1*log(dF)
% l2 = 10*lambda2*log(dist/dF)
% Pr = Prt - l1 - l2 + SH;

P_SEN = -60;

%ZeroActors = int16(zeros(15,1));
% 
% counter = 0;
% storedPacket = int16(nan(15,1));
% 
% if Pr > P_SEN
%     Actor = intVector;
%     storedPacket = intVector;
%     counter = 0;
% elseif counter < 10
%     Actor = storedPacket;
%     counter = counter + 1;
% end


%disp(storedPacket)


% persistent prev_value;
% if isempty(prev_value)
%     prev_value = int16(nan(15,1)); % Initialize to a default value
% end
% 
% if Pr > P_SEN
%     Actor = intVector;
%     prev_value = intVector;
%     counter = 0;
% elseif counter < 1
%     Actor = prev_value;
%     counter = counter + 1;
% end

Actor = intVector;
%% SNR
bandwidth = 10e6;
F = 6; % [dB] Noise figure
k = physconst('Boltzmann'); % Boltzmann állandó
T = 300; % [K] Abszolút hőmérséklet

N0 = bandwidth *k*T;
N0dbm = 10 * log10(1000*N0);
N0dbW = N0dbm - 30; 
%N0 = -99;
SNR = Pr - N0dbm;
%signalpower = Pr;s


%% Packet counter
persistent counter
if isempty(counter)
    counter = 0;
end

if (Pr > P_SEN)
    counter = counter + 1;
end

counter_out = counter;
end

== matlab function V2X_Core_SRI_coding_rate_symbol/DSRC/Subsystem6/MATLAB Function2 ==
  settings: updateMethod=DISCRETE  sampleTime=sampleTime
  data: modulated input; signal output; SNR input
function signal = PRO_error(modulated, SNR)

signal = awgn(modulated,SNR);

== matlab function V2X_Core_SRI_coding_rate_symbol/DSRC/Subsystem6/MATLAB Function3 ==
  settings: sampleTime=sampleTime
  data: input input; Actors output
function Actors = getRealValues(input) 

modulated = input;

NumActors = modulated(1,:);
Time = modulated(2,:);

ActorID = modulated(3,1);

posMultip = 10;  % 10
posX = (modulated(4,:)/posMultip);
posY = (modulated(5,:)/posMultip);
posZ = (modulated(6,:)/posMultip);

velMultip = 50;  % 50
vX = (modulated(7,:)/velMultip);
vY = (modulated(8,:)/velMultip);
vZ = (modulated(9,:)/velMultip);

rpyMultip = 50;  % 50
Roll = (modulated(10,:)/rpyMultip);
Pitch = (modulated(11,:)/rpyMultip);
Yaw = (modulated(12,:)/rpyMultip);

angvelMultip = 50;  % 50
angularVelocityX = (modulated(13,:)/angvelMultip);
angularVelocityY = (modulated(14,:)/angvelMultip);
angularVelocityZ = (modulated(15,:)/angvelMultip);

% Velocity = [vX vY vZ];
% Position = [posX posY posZ];
% AngularVelocity = [angularVelocityX; angularVelocityY; angularVelocityZ];


%Actors = [NumActors; Time; ActorID; Position; Velocity; Roll; Pitch; Yaw; AngularVelocity];
Actors = double([NumActors; Time; ActorID; posX; posY; posZ; vX; vY; vZ; Roll; Pitch; Yaw; angularVelocityX; angularVelocityY; angularVelocityZ]);


end

== matlab function V2X_Core_SRI_coding_rate_symbol/DSRC/Subsystem8/MATLAB Function1 ==
  settings: sampleTime=inherited
  data: busActors3Test1 input; Actor output int16 size=15; VehicleID input; VehicleData output Bus: Actors; EgoData input Bus: Actors; counter_out output; SNR output; Pr output
  events: trigger input RISING_EDGE_EVENT
function [Actor, VehicleData, counter_out, SNR, Pr]  = convBus2IntVector(busActors3Test1, VehicleID, EgoData)

% Data extracted from actorss bus

%ActorId = BusActors1Actors.Actors(ActorID).ActorID(1:1);
numActors = busActors3Test1.NumActors;
%time = busActors3Test1.Time;
time = busActors3Test1.Time;

ActorID = VehicleID;

posX = busActors3Test1.Actors(ActorID).Position(1:1);
posY = busActors3Test1.Actors(ActorID).Position(2:2);
posZ = busActors3Test1.Actors(ActorID).Position(3:3);
vPos = [posX posY posZ];

vX = busActors3Test1.Actors(ActorID).Velocity(1:1);
vY = busActors3Test1.Actors(ActorID).Velocity(2:2);
vZ = busActors3Test1.Actors(ActorID).Velocity(3:3);

roll = busActors3Test1.Actors(ActorID).Roll(1:1);
pitch = busActors3Test1.Actors(ActorID).Pitch(1:1);
yaw = busActors3Test1.Actors(ActorID).Yaw(1:1);


angularVelocityX = busActors3Test1.Actors(ActorID).AngularVelocity(1:1);
angularVelocityY = busActors3Test1.Actors(ActorID).AngularVelocity(2:2);
angularVelocityZ = busActors3Test1.Actors(ActorID).AngularVelocity(3:3);

VehicleData = busActors3Test1.Actors(VehicleID);


%% Converting the data

ActorID = int16(ActorID);

posMultip = 10;
posX = int16(round(posMultip*posX));
posY = int16(round(posMultip*posY));
posZ = int16(round(posMultip*posZ));

velMultip = 50;
vX = int16(round(velMultip * vX));
vY = int16(round(velMultip * vY));
vZ = int16(round(velMultip * vZ));

rpyMultip = 50;
roll = int16(round(rpyMultip * roll));
pitch = int16(round(rpyMultip * pitch));
yaw = int16(round(rpyMultip * yaw));

angvelMultip = 50;
angularVelocityX = int16(round(angvelMultip * angularVelocityX));
angularVelocityY = int16(round(angvelMultip * angularVelocityY));
angularVelocityZ = int16(round(angvelMultip * angularVelocityZ));


% Output vector
%zerosVector = zeros(9,1);

intVector = [numActors; time; ActorID; posX; posY; posZ; vX; vY; vZ; roll; pitch; yaw; angularVelocityX; angularVelocityY; angularVelocityZ];


%% Pathloss (freespace)

EgoPos = EgoData.Position;
dist = norm(vPos - EgoPos);

fc = 5.9e9;  % Carrier frequency
lambda = (physconst('LightSpeed'))/fc;

PL = fspl(dist, lambda);

Pt_dBm = 33;    % [dBm] Transmission power; maximum permissible transmit power level
Pt_dbW = Pt_dBm - 30;
sigma = rand(1) + 3.2;  % [3.7 +- 0.5] Variance of the shadowing effect in the wireless communication channel
                        % shadowing follows a log-normal random distribution
X = 2*rand(1)-1;      % random variable following a normal distribution with mean 0 and standard deviation 1
SH = sigma * X;

% h_T = 1;
% h_R = 1;
% dF =  (4*h_T*h_R)/lambda
% lambda1 = 1.61; % Pathloss exponent LOS
% lambda2 = 1.85; % Pathloss exponent NLOS

Pr = Pt_dBm - PL - SH; 

% l1 = 10*lambda1*log(dF)
% l2 = 10*lambda2*log(dist/dF)
% Pr = Prt - l1 - l2 + SH;

P_SEN = -60;

%ZeroActors = int16(zeros(15,1));
% 
% counter = 0;
% storedPacket = int16(nan(15,1));
% 
% if Pr > P_SEN
%     Actor = intVector;
%     storedPacket = intVector;
%     counter = 0;
% elseif counter < 10
%     Actor = storedPacket;
%     counter = counter + 1;
% end


%disp(storedPacket)


% persistent prev_value;
% if isempty(prev_value)
%     prev_value = int16(nan(15,1)); % Initialize to a default value
% end
% 
% if Pr > P_SEN
%     Actor = intVector;
%     prev_value = intVector;
%     counter = 0;
% elseif counter < 1
%     Actor = prev_value;
%     counter = counter + 1;
% end

Actor = intVector;
%% SNR
bandwidth = 10e6;
F = 6; % [dB] Noise figure
k = physconst('Boltzmann'); % Boltzmann állandó
T = 300; % [K] Abszolút hőmérséklet

N0 = bandwidth *k*T;
N0dbm = 10 * log10(1000*N0);
N0dbW = N0dbm - 30; 
%N0 = -99;
SNR = Pr - N0dbm;
%signalpower = Pr;s


%% Packet counter
persistent counter
if isempty(counter)
    counter = 0;
end

if (Pr > P_SEN)
    counter = counter + 1;
end

counter_out = counter;
end

== matlab function V2X_Core_SRI_coding_rate_symbol/DSRC/Subsystem8/MATLAB Function2 ==
  settings: updateMethod=DISCRETE  sampleTime=sampleTime
  data: modulated input; signal output; SNR input
function signal = PRO_error(modulated, SNR)

signal = awgn(modulated,SNR);

== matlab function V2X_Core_SRI_coding_rate_symbol/VehicleDynamic/Wheel Adapter/Camber Angle ==
  data: u input; y output
function y = fcn(u)
temp = squeeze(u(3,2:3,:));
y=atan(temp(1,:)./temp(2,:))';

== matlab function V2X_Core_SRI_coding_rate_symbol/MATLAB Function2 ==
  data: Control input; y output double size=288; Actor1 input; Actor2 input; Actor3 input; Actor4 input; Actor5 input; Actor6 input
function y = fcn(Control, Actor1, Actor2, Actor3, Actor4, Actor5, Actor6)

switch Control
    case 0
        y = Actor1;
    % case 1
    %     y = Actor2;
    % case 2
    %     y = Actor3;
    % case 3
    %     y = Actor4;
    % case 4
    %     y = Actor5;
    % case 5
    %     y = Actor6;
    otherwise
        error('Invalid control value');
end
end

== matlab function V2X_Core_SRI_coding_rate_symbol/Calculate PDR/PDR V1/MATLAB Function1 ==
  settings: sampleTime=sampleTime
  data: Vehicle_ID input; u input; y output double
function y = fcn(Vehicle_ID, u)

if isempty(u(:,Vehicle_ID)) 
    y = zeros(1,15);
else
    y = double(u(:,Vehicle_ID));
end

end

== matlab function V2X_Core_SRI_coding_rate_symbol/Calculate PDR/PDR V2/MATLAB Function ==
  settings: updateMethod=DISCRETE  sampleTime=sampleTime
  data: Tx input; PDR output; Rx input; Rx_out output; Msg_out output
function [PDR, Rx_out, Msg_out] = PDR(Tx, Rx)
    persistent N S prev_Rx
    if isempty(N) || isempty(S)
        N = 0;
        S = 0;
        prev_Rx = zeros(13,1);
    end
    if isequal(Tx, Rx) % Check if the entire vectors are the same
        N = N + 1;      % Increment the correct packet count
        prev_Rx = Rx;
        Rx_out = Rx;
        Msg_out = 1;
    else
        Rx_out = prev_Rx;
        Msg_out = 0;
    end
    S = S + 1;          % Increment the total count
    R = (N/S)*100;       % Calculate the packet delivery rate [%]
    PDR = [R; N; S];
end

== matlab function V2X_Core_SRI_coding_rate_symbol/Calculate PDR/PDR V2/MATLAB Function1 ==
  settings: sampleTime=sampleTime
  data: Vehicle_ID input; u input; y output double
function y = fcn(Vehicle_ID, u)

if isempty(u(:,Vehicle_ID)) 
    y = zeros(1,15);
else
    y = double(u(:,Vehicle_ID));
end

end

== matlab function V2X_Core_SRI_coding_rate_symbol/Calculate PDR/PDR V2/MATLAB Function2 ==
  settings: sampleTime=sampleTime
  data: Vehicle_ID input; u input; y output double
function y = fcn(Vehicle_ID, u)

if isempty(u(:,Vehicle_ID)) 
    y = zeros(1,15);
else
    y = double(u(:,Vehicle_ID));
end

end

== matlab function V2X_Core_SRI_coding_rate_symbol/Calculate PDR/PDR V2/MATLAB Function6 ==
  data: u input; y output Bus: Actors; vehicleID input
function y = fcn(u,vehicleID)

actorsCount = size(u.Actors,1);

MinusOneActor = struct(...
    'ActorID',0,...
    'Position', [0 0 0], ...
    'Velocity', [0 0 0], ...
    'Roll', 0, ...
    'Pitch', 0, ...
    'Yaw', 0, ...
    'AngularVelocity', [0 0 0]);

if actorsCount < vehicleID
    y = MinusOneActor;
else
    y = u.Actors(vehicleID);
end
end

== matlab function V2X_Core_SRI_coding_rate_symbol/Calculate PDR/PDR V3/MATLAB Function ==
  settings: updateMethod=DISCRETE  sampleTime=sampleTime
  data: Tx input; PDR output; Rx input; Rx_out output; Msg_out output
function [PDR, Rx_out, Msg_out] = PDR(Tx, Rx)
    persistent N S prev_Rx
    if isempty(N) || isempty(S)
        N = 0;
        S = 0;
        prev_Rx = zeros(13,1);
    end
    if isequal(Tx, Rx) % Check if the entire vectors are the same
        N = N + 1;      % Increment the correct packet count
        prev_Rx = Rx;
        Rx_out = Rx;
        Msg_out = 1;
    else
        Rx_out = prev_Rx;
        Msg_out = 0;
    end
    S = S + 1;          % Increment the total count
    R = (N/S)*100;       % Calculate the packet delivery rate [%]
    PDR = [R; N; S];
end

== matlab function V2X_Core_SRI_coding_rate_symbol/Calculate PDR/PDR V3/MATLAB Function1 ==
  settings: sampleTime=sampleTime
  data: Vehicle_ID input; u input; y output double
function y = fcn(Vehicle_ID, u)

if isempty(u(:,Vehicle_ID)) 
    y = zeros(1,15);
else
    y = double(u(:,Vehicle_ID));
end

end

== matlab function V2X_Core_SRI_coding_rate_symbol/Calculate PDR/PDR V3/MATLAB Function2 ==
  settings: sampleTime=sampleTime
  data: Vehicle_ID input; u input; y output double
function y = fcn(Vehicle_ID, u)

if isempty(u(:,Vehicle_ID)) 
    y = zeros(1,15);
else
    y = double(u(:,Vehicle_ID));
end

end

== matlab function V2X_Core_SRI_coding_rate_symbol/Calculate PDR/PDR V3/MATLAB Function6 ==
  data: u input; y output Bus: Actors; vehicleID input
function y = fcn(u,vehicleID)

actorsCount = size(u.Actors,1);

MinusOneActor = struct(...
    'ActorID',0,...
    'Position', [0 0 0], ...
    'Velocity', [0 0 0], ...
    'Roll', 0, ...
    'Pitch', 0, ...
    'Yaw', 0, ...
    'AngularVelocity', [0 0 0]);

if actorsCount < vehicleID
    y = MinusOneActor;
else
    y = u.Actors(vehicleID);
end
end

== matlab function V2X_Core_SRI_coding_rate_symbol/Calculate PDR/PDR V4/MATLAB Function ==
  settings: updateMethod=DISCRETE  sampleTime=sampleTime
  data: Tx input; PDR output; Rx input; Rx_out output; Msg_out output
function [PDR, Rx_out, Msg_out] = PDR(Tx, Rx)
    persistent N S prev_Rx
    if isempty(N) || isempty(S)
        N = 0;
        S = 0;
        prev_Rx = zeros(13,1);
    end
    if isequal(Tx, Rx) % Check if the entire vectors are the same
        N = N + 1;      % Increment the correct packet count
        prev_Rx = Rx;
        Rx_out = Rx;
        Msg_out = 1;
    else
        Rx_out = prev_Rx;
        Msg_out = 0;
    end
    S = S + 1;          % Increment the total count
    R = (N/S)*100;       % Calculate the packet delivery rate [%]
    PDR = [R; N; S];
end

== matlab function V2X_Core_SRI_coding_rate_symbol/Calculate PDR/PDR V1/MATLAB Function ==
  settings: updateMethod=DISCRETE  sampleTime=sampleTime
  data: Tx input; PDR output; Rx input; Rx_out output; Msg_out output; c_out output
function [PDR, Rx_out, Msg_out, c_out] = PDR(Tx, Rx)
    persistent N S prev_Rx counter
    if isempty(N) || isempty(S)
        N = 0;
        S = 0;
        counter = 0;
        prev_Rx = zeros(13,1);
    end
    if isequal(Tx, Rx) % Check if the entire vectors are the same
        N = N + 1;      % Increment the correct packet count
        counter = 0;
        % if counter < 20
        %     prev_Rx = Rx;
        % else
        %     prev_Rx = zeros(13,1);
        % end
        prev_Rx = Rx;
        Rx_out = Rx;
        Msg_out = 1;
    else
        Rx_out = prev_Rx;
        counter = counter + 1;
        Msg_out = 0;
    end
    S = S + 1;          % Increment the total count
    R = (N/S)*100;       % Calculate the packet delivery rate [%]
    PDR = [R; N; S];
    c_out = counter;
end

== matlab function V2X_Core_SRI_coding_rate_symbol/Calculate PDR/PDR V1/MATLAB Function2 ==
  settings: sampleTime=sampleTime
  data: Vehicle_ID input; u input; y output double
function y = fcn(Vehicle_ID, u)

if isempty(u(:,Vehicle_ID)) 
    y = zeros(1,15);
else
    y = double(u(:,Vehicle_ID));
end

end

== matlab function V2X_Core_SRI_coding_rate_symbol/Calculate PDR/PDR V1/MATLAB Function6 ==
  data: u input; y output Bus: Actors; vehicleID input
function y = fcn(u,vehicleID)

actorsCount = size(u.Actors,1);

MinusOneActor = struct(...
    'ActorID',0,...
    'Position', [0 0 0], ...
    'Velocity', [0 0 0], ...
    'Roll', 0, ...
    'Pitch', 0, ...
    'Yaw', 0, ...
    'AngularVelocity', [0 0 0]);

if actorsCount < vehicleID
    y = MinusOneActor;
else
    y = u.Actors(vehicleID);
end
end

== matlab function V2X_Core_SRI_coding_rate_symbol/Calculate PDR/PDR V4/MATLAB Function1 ==
  settings: sampleTime=sampleTime
  data: Vehicle_ID input; u input; y output double
function y = fcn(Vehicle_ID, u)

if isempty(u(:,Vehicle_ID)) 
    y = zeros(1,15);
else
    y = double(u(:,Vehicle_ID));
end

end

== matlab function V2X_Core_SRI_coding_rate_symbol/Calculate PDR/PDR V4/MATLAB Function2 ==
  settings: sampleTime=sampleTime
  data: Vehicle_ID input; u input; y output double
function y = fcn(Vehicle_ID, u)

if isempty(u(:,Vehicle_ID)) 
    y = zeros(1,15);
else
    y = double(u(:,Vehicle_ID));
end

end

== matlab function V2X_Core_SRI_coding_rate_symbol/Calculate PDR/PDR V4/MATLAB Function6 ==
  data: u input; y output Bus: Actors; vehicleID input
function y = fcn(u,vehicleID)

actorsCount = size(u.Actors,1);

MinusOneActor = struct(...
    'ActorID',0,...
    'Position', [0 0 0], ...
    'Velocity', [0 0 0], ...
    'Roll', 0, ...
    'Pitch', 0, ...
    'Yaw', 0, ...
    'AngularVelocity', [0 0 0]);

if actorsCount < vehicleID
    y = MinusOneActor;
else
    y = u.Actors(vehicleID);
end
end
